simulink model "two_parallel_full_model_simscape"  (R2023b)
settings: Solver=ode1be  StartTime=0.0  StopTime=simlength  FixedStep=ts_sim  MaxStep=ts_sim
undefined symbols (not defined in the file): fclock, fPWM_INV, fPWM_ZVS, gate_nominal_voltage, I_FS, Iout_dc_nom, ki_i_inv, ki_i_zvs, ki_v_inv, ki_v_zvs, kp_i_inv, kp_i_zvs, kp_v_inv, kp_v_zvs, LFi_dc, LFu_ac, magnitude, n10, omega_grid, RCFu_dc, RLFi_dc, RLFu_ac, tc, Tc, tPWM_ZVS, ts_afe, ts_inv, ts_zvs, ugrid_factor, Ugrid_phase_normalization_factor, un_eta_pu, un_xi_pu, up_xi_pu, v1_trafo, v2_trafo, V_FS, Vout_dc_nom
libraries: fl_lib x142, nesl_utility x55, single_phase_transformer_lib x4
(part 1 of 4)
settings Model: SimulationMode=accelerator  Creator=LTNBDA  LastModifiedBy=dbagn
settings SolverCC: ZeroCrossControl=EnableAll  ZeroCrossAlgorithm=Adaptive  AlgebraicLoopSolver=TrustRegion  SolverResetMethod=Robust  AutoInsertRateTranBlk=on
settings DataIOCC: LimitDataPoints=on  MaxDataPoints=1  SaveFormat=Array  SignalLoggingSaveFormat=ModelDataLogs  SaveOutput=off  SignalLogging=off  DSMLogging=off  SaveTime=off  ReturnWorkspaceOutputs=off
settings OptimizationCC: ExpressionDepthLimit=2147483647  InitFltsAndDblsToZero=on  EfficientMapNaN2IntZero=off  LifeSpan=inf
settings DebuggingCC: SaveWithParameterizedLinksMsg=none  UnderspecifiedInitializationDetection=Classic  MergeDetectMultiDrivingBlocksExec=none  SignalResolutionControl=TryResolveAllWithWarning  SolverPrmCheckMsg=warning  MultiTaskDSMMsg=warning  MultiTaskCondExecSysMsg=none  MultiTaskRateTransMsg=warning  FcnCallInpInsideContextMsg=warning  StateNameClashWarn=warning  SFUnexpectedBacktrackingDiag=warning  SFNoUnconditionalDefaultTransitionDiag=warning  ArithmeticOperatorsInVariantConditions=warning
settings HardwareCC: ProdBitPerLong=64  ProdLargestAtomicFloat=None  ProdIntDivRoundTo=Undefined  ProdEndianess=Unspecified  ProdHWDeviceType=Generic->64-bit Embedded Processor (LP64)  TargetBitPerPointer=64  TargetBitPerSizeT=64  TargetBitPerPtrDiffT=64  TargetLongLongMode=on  TargetIntDivRoundTo=Zero  TargetEndianess=LittleEndian  TargetWordSize=64  TargetHWDeviceType=MATLAB Host  ProdEqTarget=off
settings ModelReferenceCC: EnableRefExpFcnMdlSchedulingChecks=on  PropagateSignalLabelsOutOfModel=off
settings SFSimCC: SimUseLocalCustomCode=off  CustomCodeUndefinedFunction=UseInterfaceOnly
settings RTWCC: RTWUseLocalCustomCode=off
settings CodeAppCC: MaxIdLength=128  StateflowObjectComments=on
settings GRTTargetCC: TargetLangStandard=C89/C90 (ANSI)  CombineOutputUpdateFcns=off  GRTInterface=on
settings ConfigComp: CovMetricSettings=dw  CovSaveCumulativeToWorkspaceVar=on  CovSaveSingleToWorkspaceVar=on  CovExternalEMLEnable=off
settings SimscapeCC: SimscapeNormalizeSystem=off

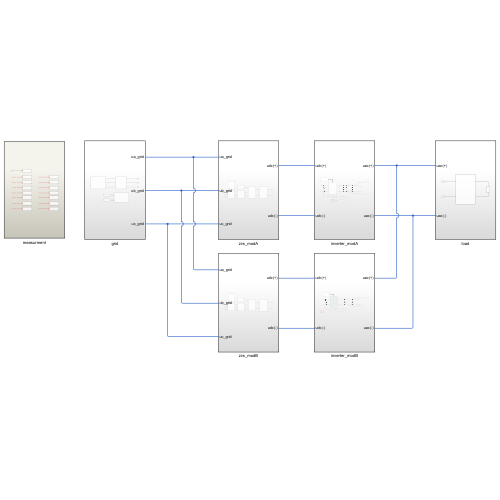
[thumbnail: Simulink's stored preview of the top-level diagram]
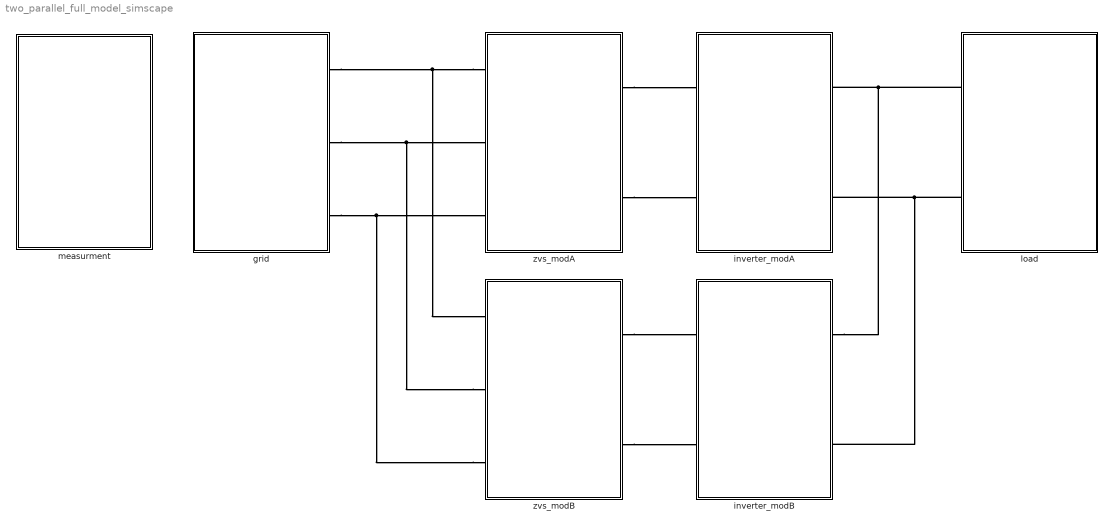
== system two_parallel_full_model_simscape ==
  grid : Subsystem
  inverter_modA : Subsystem
  inverter_modB : Subsystem
  load : Subsystem
  measurment : Subsystem
  zvs_modA : Subsystem
  zvs_modB : Subsystem
  connections:
  load/LConn1 -- inverter_modB/RConn1 -- inverter_modA/RConn1
  load/LConn2 -- inverter_modB/RConn2 -- inverter_modA/RConn2
  zvs_modA/LConn1 -- grid/RConn1 -- zvs_modB/LConn1
  zvs_modB/LConn2 -- grid/RConn2 -- zvs_modA/LConn2
  zvs_modB/LConn3 -- grid/RConn3 -- zvs_modA/LConn3
  zvs_modA/RConn2 -- inverter_modA/LConn2
  zvs_modA/RConn1 -- inverter_modA/LConn1
  zvs_modB/RConn1 -- inverter_modB/LConn1
  zvs_modB/RConn2 -- inverter_modB/LConn2

== system two_parallel_full_model_simscape/grid ==
  grid_emulator : Subsystem
  instantaneus_power : Subsystem
  threephase_vi_measures : Subsystem
  ua_grid : PMIOPort  Side=Right
  ub_grid : PMIOPort  Port=2  Side=Right
  uc_grid : PMIOPort  Port=3  Side=Right
  wires:
  [vg_abc] -> instantaneus_power/1(Vline)
  [ig_abc] -> instantaneus_power/2(Iline)
  connections:
  threephase_vi_measures/LConn3 -- grid_emulator/RConn3
  threephase_vi_measures/LConn2 -- grid_emulator/RConn2
  threephase_vi_measures/RConn1 -- ua_grid/RConn1
  threephase_vi_measures/LConn1 -- grid_emulator/RConn1
  threephase_vi_measures/RConn3 -- uc_grid/RConn1
  threephase_vi_measures/RConn2 -- ub_grid/RConn1

== system two_parallel_full_model_simscape/inverter_modA ==
  1/Ti3 : Gain  Gain=1/V_FS  SaturateOnIntegerOverflow=on  OutDataTypeStr=Inherit: Same as input  ParamDataTypeStr=Inherit: Same as input
  CFu_ac : fl_lib/Electrical/Electrical Elements/Capacitor  c=CFu_ac F  r=RCFu_ac Ohm  g=0 1/Ohm  i_specify=off  i_priority=None  i=0 A  i_nominal_specify=off  i_nominal_unit=A  i_nominal_value=1  v_specify=off  v_priority=None  v=0 V  v_nominal_specify=off  v_nominal_unit=V  v_nominal_value=1  vc_specify=off  vc_priority=High  vc=0 V  vc_nominal_specify=off  vc_nominal_unit=V  vc_nominal_value=1
  Current Sensor : fl_lib/Electrical/Electrical Sensors/Current Sensor
  Inductor1 : fl_lib/Electrical/Electrical Elements/Inductor  l=Lp H  r=0 Ohm  g=1e-9 1/Ohm  i_specify=off  i_priority=None  i=0 A  i_nominal_specify=off  i_nominal_unit=A  i_nominal_value=1  v_specify=off  v_priority=None  v=0 V  v_nominal_specify=off  v_nominal_unit=V  v_nominal_value=1  i_L_specify=off  i_L_priority=High  i_L=0 A  i_L_nominal_specify=off  i_L_nominal_unit=A  i_L_nominal_value=1
  Inductor2 : fl_lib/Electrical/Electrical Elements/Inductor  l=Lp H  r=0 Ohm  g=1e-9 1/Ohm  i_specify=off  i_priority=None  i=0 A  i_nominal_specify=off  i_nominal_unit=A  i_nominal_value=1  v_specify=off  v_priority=None  v=0 V  v_nominal_specify=off  v_nominal_unit=V  v_nominal_value=1  i_L_specify=off  i_L_priority=High  i_L=0 A  i_L_nominal_specify=off  i_L_nominal_unit=A  i_L_nominal_value=1
  LFu_ac_1 : fl_lib/Electrical/Electrical Elements/Inductor  l=LFu_ac/2 H  r=RLFu_ac/2 Ohm  g=0 1/Ohm  i_specify=off  i_priority=None  i=0 A  i_nominal_specify=off  i_nominal_unit=A  i_nominal_value=1  v_specify=off  v_priority=None  v=0 V  v_nominal_specify=off  v_nominal_unit=V  v_nominal_value=1  i_L_specify=off  i_L_priority=High  i_L=0 A  i_L_nominal_specify=off  i_L_nominal_unit=A  i_L_nominal_value=1
  LFu_ac_2 : fl_lib/Electrical/Electrical Elements/Inductor  l=LFu_ac/2 H  r=RLFu_ac/2 Ohm  g=0 1/Ohm  i_specify=off  i_priority=None  i=0 A  i_nominal_specify=off  i_nominal_unit=A  i_nominal_value=1  v_specify=off  v_priority=None  v=0 V  v_nominal_specify=off  v_nominal_unit=V  v_nominal_value=1  i_L_specify=off  i_L_priority=High  i_L=0 A  i_L_nominal_specify=off  i_L_nominal_unit=A  i_L_nominal_value=1
  Resistor : fl_lib/Electrical/Electrical Elements/Resistor  R=10e3 Ohm  i_specify=off  i_priority=None  i=0 A  i_nominal_specify=off  i_nominal_unit=A  i_nominal_value=1  v_specify=off  v_priority=None  v=0 V  v_nominal_specify=off  v_nominal_unit=V  v_nominal_value=1
  Voltage Sensor : fl_lib/Electrical/Electrical Sensors/Voltage Sensor
  Voltage Sensor1 : fl_lib/Electrical/Electrical Sensors/Voltage Sensor
  Zero-Order Hold2 : ZeroOrderHold  SampleTime=ts_zvs
  iph : nesl_utility/PS-Simulink Converter  PhysicalDomain=network_engine_domain  SubClassName=ps_output  LeftPortType=input  RightPortType=output  PseudoPeriodic=off  Frequencies=[]  VectorFormat=1-D array  Unit=A  AffineConversion=off
  phase_gen : Subsystem
  single phase inverter : Subsystem
      settings: PortSchema="{\"entries\":[{\"content\":{\"sides\":[{\"content\":{\"connectorIds\":[\"LConn1\",\"LConn2\"]},\"type\":\"ConnectorPlacement.EquallySpacedRectSide\",\"uuid\":\"4fcf4fea-d38f-431b-8a91-be3ce9782faf\"},{\"content\":{\"connectorIds\":[\"RConn1\",\"RConn2\"],\"side\":\"RIGHT\"},\"type\":\"ConnectorPlacement.EquallySpacedRectSide\",\"uuid\":\"0aa56277-92e9-4e3b-84c7-43398254a4d8\"},{\"content\":{\"connectorIds\":[\"In1\"],\"side\":\"TOP\"},\"type\":\"ConnectorPlacement.EquallySpacedRectSide\",\"uuid\":\"5cd150dc-bcaf-4cd7-b2a8-3db203726730\"}]},\"type\":\"ConnectorPlacement.EquallySpacedConnector\",\"uuid\":\"bf8194c4-c327-4d40-bea4-f1e7617f80b4\"}],\"packageUris\":[\"http://schema.mathworks.com/mf0/Connector/R2020b\"],\"version\":\"1.0\"}"
  single phase inverter control : Subsystem
  uph : nesl_utility/PS-Simulink Converter  PhysicalDomain=network_engine_domain  SubClassName=ps_output  LeftPortType=input  RightPortType=output  PseudoPeriodic=off  Frequencies=[]  VectorFormat=1-D array  Unit=V  AffineConversion=off
  uph1 : nesl_utility/PS-Simulink Converter  PhysicalDomain=network_engine_domain  SubClassName=ps_output  LeftPortType=input  RightPortType=output  PseudoPeriodic=off  Frequencies=[]  VectorFormat=1-D array  Unit=V  AffineConversion=off
  uac(+) : PMIOPort  Side=Right
  uac(-) : PMIOPort  Port=2  Side=Right
  udc(+) : PMIOPort  Port=3  Side=Left
  udc(-) : PMIOPort  Port=4  Side=Left
  tag scope: dclink_voltage_modA=global, inverter_current_output_modA=global, inverter_voltager_output_modA=global, phase_synch_modA=global
  wires:
  Zero-Order Hold2/1 -> 1/Ti3/1
  1/Ti3/1 -> [dclink_voltage_modA]
  single phase inverter control/1(gate_commands) -> single phase inverter/1(gate_commands)
  uph/1 -> Zero-Order Hold2/1  "uph"
  iph/1 -> [inverter_current_output_modA]  "iph"
  uph1/1 -> [inverter_voltager_output_modA]  "uph"
  phase_gen/1(emu_phase) -> [phase_synch_modA]
  connections:
  single phase inverter/RConn2 -- Voltage Sensor/RConn2 -- udc(-)/RConn1
  single phase inverter/RConn1 -- Voltage Sensor/LConn1 -- udc(+)/RConn1
  LFu_ac_1/LConn1 -- single phase inverter/LConn1
  Inductor1/RConn1 -- Voltage Sensor1/LConn1 -- Current Sensor/LConn1
  single phase inverter/LConn2 -- LFu_ac_2/RConn1
  LFu_ac_2/LConn1 -- Inductor2/LConn1 -- Resistor/RConn1 -- CFu_ac/RConn1
  Voltage Sensor/RConn1 -- uph/LConn1
  Voltage Sensor1/RConn1 -- uph1/LConn1
  Current Sensor/RConn1 -- iph/LConn1
  Voltage Sensor1/RConn2 -- Inductor2/RConn1 -- uac(-)/RConn1
  CFu_ac/LConn1 -- Inductor1/LConn1 -- Resistor/LConn1 -- LFu_ac_1/RConn1
  Current Sensor/RConn2 -- uac(+)/RConn1

== system two_parallel_full_model_simscape/inverter_modB ==
  1/Ti3 : Gain  Gain=1/V_FS  SaturateOnIntegerOverflow=on  OutDataTypeStr=Inherit: Same as input  ParamDataTypeStr=Inherit: Same as input
  CFu_ac : fl_lib/Electrical/Electrical Elements/Capacitor  c=CFu_ac F  r=RCFu_ac Ohm  g=0 1/Ohm  i_specify=off  i_priority=None  i=0 A  i_nominal_specify=off  i_nominal_unit=A  i_nominal_value=1  v_specify=off  v_priority=None  v=0 V  v_nominal_specify=off  v_nominal_unit=V  v_nominal_value=1  vc_specify=off  vc_priority=High  vc=0 V  vc_nominal_specify=off  vc_nominal_unit=V  vc_nominal_value=1
  Current Sensor : fl_lib/Electrical/Electrical Sensors/Current Sensor
  Inductor : fl_lib/Electrical/Electrical Elements/Inductor  l=Lp H  r=0 Ohm  g=1e-9 1/Ohm  i_specify=off  i_priority=None  i=0 A  i_nominal_specify=off  i_nominal_unit=A  i_nominal_value=1  v_specify=off  v_priority=None  v=0 V  v_nominal_specify=off  v_nominal_unit=V  v_nominal_value=1  i_L_specify=off  i_L_priority=High  i_L=0 A  i_L_nominal_specify=off  i_L_nominal_unit=A  i_L_nominal_value=1
  Inductor1 : fl_lib/Electrical/Electrical Elements/Inductor  l=Lp H  r=0 Ohm  g=1e-9 1/Ohm  i_specify=off  i_priority=None  i=0 A  i_nominal_specify=off  i_nominal_unit=A  i_nominal_value=1  v_specify=off  v_priority=None  v=0 V  v_nominal_specify=off  v_nominal_unit=V  v_nominal_value=1  i_L_specify=off  i_L_priority=High  i_L=0 A  i_L_nominal_specify=off  i_L_nominal_unit=A  i_L_nominal_value=1
  LFu_ac_1 : fl_lib/Electrical/Electrical Elements/Inductor  l=LFu_ac/2 H  r=RLFu_ac/2 Ohm  g=0 1/Ohm  i_specify=off  i_priority=None  i=0 A  i_nominal_specify=off  i_nominal_unit=A  i_nominal_value=1  v_specify=off  v_priority=None  v=0 V  v_nominal_specify=off  v_nominal_unit=V  v_nominal_value=1  i_L_specify=off  i_L_priority=High  i_L=0 A  i_L_nominal_specify=off  i_L_nominal_unit=A  i_L_nominal_value=1
  LFu_ac_2 : fl_lib/Electrical/Electrical Elements/Inductor  l=LFu_ac/2 H  r=RLFu_ac/2 Ohm  g=0 1/Ohm  i_specify=off  i_priority=None  i=0 A  i_nominal_specify=off  i_nominal_unit=A  i_nominal_value=1  v_specify=off  v_priority=None  v=0 V  v_nominal_specify=off  v_nominal_unit=V  v_nominal_value=1  i_L_specify=off  i_L_priority=High  i_L=0 A  i_L_nominal_specify=off  i_L_nominal_unit=A  i_L_nominal_value=1
  Resistor : fl_lib/Electrical/Electrical Elements/Resistor  R=10e3 Ohm  i_specify=off  i_priority=None  i=0 A  i_nominal_specify=off  i_nominal_unit=A  i_nominal_value=1  v_specify=off  v_priority=None  v=0 V  v_nominal_specify=off  v_nominal_unit=V  v_nominal_value=1
  Voltage Sensor : fl_lib/Electrical/Electrical Sensors/Voltage Sensor
  Voltage Sensor1 : fl_lib/Electrical/Electrical Sensors/Voltage Sensor
  Zero-Order Hold2 : ZeroOrderHold  SampleTime=ts_zvs
  iph : nesl_utility/PS-Simulink Converter  PhysicalDomain=network_engine_domain  SubClassName=ps_output  LeftPortType=input  RightPortType=output  PseudoPeriodic=off  Frequencies=[]  VectorFormat=1-D array  Unit=A  AffineConversion=off
  phase_gen : Subsystem
  single phase inverter : Subsystem
      settings: PortSchema="{\"entries\":[{\"content\":{\"sides\":[{\"content\":{\"connectorIds\":[\"LConn1\",\"LConn2\"]},\"type\":\"ConnectorPlacement.EquallySpacedRectSide\",\"uuid\":\"4fcf4fea-d38f-431b-8a91-be3ce9782faf\"},{\"content\":{\"connectorIds\":[\"RConn1\",\"RConn2\"],\"side\":\"RIGHT\"},\"type\":\"ConnectorPlacement.EquallySpacedRectSide\",\"uuid\":\"0aa56277-92e9-4e3b-84c7-43398254a4d8\"},{\"content\":{\"connectorIds\":[\"In1\"],\"side\":\"TOP\"},\"type\":\"ConnectorPlacement.EquallySpacedRectSide\",\"uuid\":\"5cd150dc-bcaf-4cd7-b2a8-3db203726730\"}]},\"type\":\"ConnectorPlacement.EquallySpacedConnector\",\"uuid\":\"bf8194c4-c327-4d40-bea4-f1e7617f80b4\"}],\"packageUris\":[\"http://schema.mathworks.com/mf0/Connector/R2020b\"],\"version\":\"1.0\"}"
  single phase inverter control : Subsystem
  uph : nesl_utility/PS-Simulink Converter  PhysicalDomain=network_engine_domain  SubClassName=ps_output  LeftPortType=input  RightPortType=output  PseudoPeriodic=off  Frequencies=[]  VectorFormat=1-D array  Unit=V  AffineConversion=off
  uph1 : nesl_utility/PS-Simulink Converter  PhysicalDomain=network_engine_domain  SubClassName=ps_output  LeftPortType=input  RightPortType=output  PseudoPeriodic=off  Frequencies=[]  VectorFormat=1-D array  Unit=V  AffineConversion=off
  uac(+) : PMIOPort  Side=Right
  uac(-) : PMIOPort  Port=2  Side=Right
  udc(+) : PMIOPort  Port=3  Side=Left
  udc(-) : PMIOPort  Port=4  Side=Left
  tag scope: dclink_voltage_modB=global, inverter_current_output_modB=global, inverter_voltager_output_modB=global, phase_synch_modB=global
  wires:
  uph1/1 -> [inverter_voltager_output_modB]  "uph"
  iph/1 -> [inverter_current_output_modB]  "iph"
  uph/1 -> Zero-Order Hold2/1  "uph"
  single phase inverter control/1(gate_commands) -> single phase inverter/1(gate_commands)
  1/Ti3/1 -> [dclink_voltage_modB]
  Zero-Order Hold2/1 -> 1/Ti3/1
  [gamma] -> [phase_synch_modB]
  connections:
  Current Sensor/RConn1 -- iph/LConn1
  Voltage Sensor1/RConn1 -- uph1/LConn1
  Voltage Sensor/RConn1 -- uph/LConn1
  Voltage Sensor1/RConn2 -- Inductor1/RConn1 -- uac(-)/RConn1
  single phase inverter/LConn2 -- LFu_ac_2/RConn1
  Inductor/RConn1 -- Voltage Sensor1/LConn1 -- Current Sensor/LConn1
  LFu_ac_1/LConn1 -- single phase inverter/LConn1
  Voltage Sensor/LConn1 -- single phase inverter/RConn1 -- udc(+)/RConn1
  Voltage Sensor/RConn2 -- udc(-)/RConn1 -- single phase inverter/RConn2
  Resistor/LConn1 -- CFu_ac/LConn1 -- LFu_ac_1/RConn1 -- Inductor/LConn1
  Resistor/RConn1 -- Inductor1/LConn1 -- LFu_ac_2/LConn1 -- CFu_ac/RConn1
  Current Sensor/RConn2 -- uac(+)/RConn1

== system two_parallel_full_model_simscape/load ==
  RL-load : fl_lib/Electrical/Electrical Elements/Inductor  l=Lload H  r=Rload Ohm  g=0 1/Ohm  i_specify=off  i_priority=None  i=0 A  i_nominal_specify=off  i_nominal_unit=A  i_nominal_value=1  v_specify=off  v_priority=None  v=0 V  v_nominal_specify=off  v_nominal_unit=V  v_nominal_value=1  i_L_specify=off  i_L_priority=High  i_L=0 A  i_L_nominal_specify=off  i_L_nominal_unit=A  i_L_nominal_value=1
  single_phase_ui_measure : Subsystem
  uac(+) : PMIOPort  Side=Left
  uac(-) : PMIOPort  Port=2  Side=Left
  connections:
  single_phase_ui_measure/LConn1 -- uac(+)/RConn1
  uac(-)/RConn1 -- single_phase_ui_measure/LConn2
  single_phase_ui_measure/RConn1 -- RL-load/LConn1
  RL-load/RConn1 -- single_phase_ui_measure/RConn2

== system two_parallel_full_model_simscape/measurment ==
  Clock : Clock
  To Workspace1 : ToWorkspace  VariableName=t  SampleTime=tc
      settings: MaxDataPoints=Nc
  To Workspace10 : ToWorkspace  Commented=on  VariableName=vi_CFu_ac  SampleTime=tc
      settings: MaxDataPoints=Nc
  To Workspace11 : ToWorkspace  Commented=on  VariableName=vi_LFu_ac  SampleTime=tc
      settings: MaxDataPoints=Nc
  To Workspace12 : ToWorkspace  Commented=on  VariableName=vi_LFi_dc  SampleTime=tc
      settings: MaxDataPoints=Nc
  To Workspace13 : ToWorkspace  Commented=on  VariableName=vi_Ls  SampleTime=tc
      settings: MaxDataPoints=Nc
  To Workspace14 : ToWorkspace  Commented=on  VariableName=vi_CFi_dc  SampleTime=tc
      settings: MaxDataPoints=Nc
  To Workspace15 : ToWorkspace  Commented=on  VariableName=i_d_rect  SampleTime=tc
      settings: MaxDataPoints=Nc
  To Workspace2 : ToWorkspace  Commented=on  VariableName=vi_RCFu_dc  SampleTime=tc
      settings: MaxDataPoints=Nc
  To Workspace3 : ToWorkspace  Commented=on  VariableName=vi_LFu_dc  SampleTime=tc
      settings: MaxDataPoints=Nc
  To Workspace4 : ToWorkspace  Commented=on  VariableName=vi_Cs  SampleTime=tc
      settings: MaxDataPoints=Nc
  To Workspace5 : ToWorkspace  Commented=on  VariableName=vi_load  SampleTime=tc
      settings: MaxDataPoints=Nc
  To Workspace6 : ToWorkspace  Commented=on  VariableName=vi_CFu_dc  SampleTime=tc
      settings: MaxDataPoints=Nc
  To Workspace7 : ToWorkspace  Commented=on  VariableName=vdc_in  SampleTime=tc
      settings: MaxDataPoints=Nc
  To Workspace8 : ToWorkspace  Commented=on  VariableName=Isnubber_H  SampleTime=tc
      settings: MaxDataPoints=Nc
  To Workspace9 : ToWorkspace  Commented=on  VariableName=Isnubber_Rect1  SampleTime=tc
      settings: MaxDataPoints=Nc
  wires:
  Clock/1 -> To Workspace1/1
  ? -> To Workspace3/1
  ? -> To Workspace6/1
  ? -> To Workspace2/1
  ? -> To Workspace4/1
  ? -> To Workspace5/1
  ? -> To Workspace7/1
  ? -> To Workspace8/1
  ? -> To Workspace9/1
  ? -> To Workspace11/1
  ? -> To Workspace10/1
  ? -> To Workspace12/1
  ? -> To Workspace13/1
  ? -> To Workspace14/1
  ? -> To Workspace15/1

== system two_parallel_full_model_simscape/zvs_modA ==
  dc/dc with galvanic isolation : Subsystem
  grid_rectifier : Subsystem
  measurment : Subsystem  Commented=on
  single_phase_ui_measure : Subsystem
  three_phase_vi_measures : Subsystem
  zvs_ctrl : Subsystem
  ua_grid : PMIOPort  Side=Left
  ub_grid : PMIOPort  Port=2  Side=Left
  uc_grid : PMIOPort  Port=3  Side=Left
  udc(+) : PMIOPort  Port=4  Side=Right
  udc(-) : PMIOPort  Port=5  Side=Right
  wires:
  zvs_ctrl/1(gate_commands) -> dc/dc with galvanic isolation/1(gate_commands)
  connections:
  grid_rectifier/LConn1 -- three_phase_vi_measures/RConn1
  grid_rectifier/LConn2 -- three_phase_vi_measures/RConn2
  grid_rectifier/LConn3 -- three_phase_vi_measures/RConn3
  ua_grid/RConn1 -- three_phase_vi_measures/LConn1
  ub_grid/RConn1 -- three_phase_vi_measures/LConn2
  uc_grid/RConn1 -- three_phase_vi_measures/LConn3
  dc/dc with galvanic isolation/LConn1 -- grid_rectifier/RConn1
  dc/dc with galvanic isolation/LConn2 -- grid_rectifier/RConn2
  dc/dc with galvanic isolation/RConn1 -- single_phase_ui_measure/LConn1
  dc/dc with galvanic isolation/RConn2 -- single_phase_ui_measure/LConn2
  udc(+)/RConn1 -- single_phase_ui_measure/RConn1
  udc(-)/RConn1 -- single_phase_ui_measure/RConn2

== system two_parallel_full_model_simscape/zvs_modB ==
  dc/dc with galvanic isolation : Subsystem
  grid_rectifier : Subsystem
  measurment : Subsystem  Commented=on
  single_phase_ui_measure : Subsystem
  three_phase_vi_measures : Subsystem
  zvs_ctrl : Subsystem
  ua_grid : PMIOPort  Side=Left
  ub_grid : PMIOPort  Port=2  Side=Left
  uc_grid : PMIOPort  Port=3  Side=Left
  udc(+) : PMIOPort  Port=4  Side=Right
  udc(-) : PMIOPort  Port=5  Side=Right
  wires:
  zvs_ctrl/1(gate_commands) -> dc/dc with galvanic isolation/1(gate_commands)
  connections:
  udc(-)/RConn1 -- single_phase_ui_measure/RConn2
  udc(+)/RConn1 -- single_phase_ui_measure/RConn1
  dc/dc with galvanic isolation/RConn2 -- single_phase_ui_measure/LConn2
  dc/dc with galvanic isolation/RConn1 -- single_phase_ui_measure/LConn1
  dc/dc with galvanic isolation/LConn2 -- grid_rectifier/RConn2
  dc/dc with galvanic isolation/LConn1 -- grid_rectifier/RConn1
  uc_grid/RConn1 -- three_phase_vi_measures/LConn3
  ub_grid/RConn1 -- three_phase_vi_measures/LConn2
  ua_grid/RConn1 -- three_phase_vi_measures/LConn1
  grid_rectifier/LConn3 -- three_phase_vi_measures/RConn3
  grid_rectifier/LConn2 -- three_phase_vi_measures/RConn2
  grid_rectifier/LConn1 -- three_phase_vi_measures/RConn1

== system two_parallel_full_model_simscape/grid/grid_emulator ==
  Controlled Voltage Source : fl_lib/Electrical/Electrical Sources/Controlled Voltage Source
  Controlled Voltage Source1 : fl_lib/Electrical/Electrical Sources/Controlled Voltage Source
  Controlled Voltage Source2 : fl_lib/Electrical/Electrical Sources/Controlled Voltage Source
  Electrical Reference : fl_lib/Electrical/Electrical Elements/Electrical Reference
  Ld2_grid_1 : fl_lib/Electrical/Electrical Elements/Inductor  l=60e-6 H  r=5e-3 Ohm  g=1e-9 1/Ohm  i_specify=on  i_priority=High  i=0 A  i_nominal_specify=off  i_nominal_unit=A  i_nominal_value=1  v_specify=off  v_priority=None  v=0 V  v_nominal_specify=off  v_nominal_unit=V  v_nominal_value=1  i_L_specify=off  i_L_priority=High  i_L=0 A  i_L_nominal_specify=off  i_L_nominal_unit=A  i_L_nominal_value=1
  Ld2_grid_2 : fl_lib/Electrical/Electrical Elements/Inductor  l=60e-6 H  r=5e-3 Ohm  g=1e-9 1/Ohm  i_specify=on  i_priority=High  i=0 A  i_nominal_specify=off  i_nominal_unit=A  i_nominal_value=1  v_specify=off  v_priority=None  v=0 V  v_nominal_specify=off  v_nominal_unit=V  v_nominal_value=1  i_L_specify=off  i_L_priority=High  i_L=0 A  i_L_nominal_specify=off  i_L_nominal_unit=A  i_L_nominal_value=1
  Ld2_grid_3 : fl_lib/Electrical/Electrical Elements/Inductor  l=60e-6 H  r=5e-3 Ohm  g=1e-9 1/Ohm  i_specify=on  i_priority=High  i=0 A  i_nominal_specify=off  i_nominal_unit=A  i_nominal_value=1  v_specify=off  v_priority=None  v=0 V  v_nominal_specify=off  v_nominal_unit=V  v_nominal_value=1  i_L_specify=off  i_L_priority=High  i_L=0 A  i_L_nominal_specify=off  i_L_nominal_unit=A  i_L_nominal_value=1
  Simulink-PS Converter : nesl_utility/Simulink-PS Converter  PhysicalDomain=network_engine_domain  SubClassName=ps_input  LeftPortType=input  RightPortType=output  PseudoPeriodic=off  Frequencies=[]  NoiseDistribution=none  NoiseParameters=[]  Unit=V  AffineConversion=on  FilteringAndDerivatives=provide  SimscapeFilterOrder=1  InputFilterTimeConstant=0.001  UdotUserProvided=0
  Simulink-PS Converter1 : nesl_utility/Simulink-PS Converter  PhysicalDomain=network_engine_domain  SubClassName=ps_input  LeftPortType=input  RightPortType=output  PseudoPeriodic=off  Frequencies=[]  NoiseDistribution=none  NoiseParameters=[]  Unit=V  AffineConversion=on  FilteringAndDerivatives=provide  SimscapeFilterOrder=1  InputFilterTimeConstant=0.001  UdotUserProvided=0
  Simulink-PS Converter2 : nesl_utility/Simulink-PS Converter  PhysicalDomain=network_engine_domain  SubClassName=ps_input  LeftPortType=input  RightPortType=output  PseudoPeriodic=off  Frequencies=[]  NoiseDistribution=none  NoiseParameters=[]  Unit=V  AffineConversion=on  FilteringAndDerivatives=provide  SimscapeFilterOrder=1  InputFilterTimeConstant=0.001  UdotUserProvided=0
  Solver Configuration : nesl_utility/Solver Configuration  PhysicalDomain=network_engine_domain  SubClassName=solver  LeftPortType=input  RightPortType=generic  Tones=[]  Harmonics=[]  SimulateNoise=off  Profile=off  UseLocalSampling=off  EnableSwitchedLinearOptims=on  FrequencyDomain=off  UseCCode=off  RelTol=0.001  AbsTol=0.001  MinStep=1e-09  ToWorkspace=off  RevertToSquareIcSolve=off  NumHomotopyIterations=100  PhasorMode=off  PhasorModeNumHarmonics=1  ConsistencySolver=NEWTON_FTOL  IndexReductionMethod=DerivativeReplacement  DoDC=on  ResidualTolerance=1e-09  ConsistencyTolSource=GLOBAL  ConsistencyAbsTol=0.001  ConsistencyRelTol=0.001  ConsistencyTolFactor=0.001  UseLocalSolver=on  LocalSolverChoice=NE_BACKWARD_EULER_ADVANCER  ResolveIndetEquations=on  FunctionEvalNumThread=1  LocalSolverSampleTime=ts_sim  DoFixedCost=on  MaxNonlinIter=3  MaxModeIter=2  ComputeImpulses=off  ImpulseIterations=2  LinearAlgebra=auto  LinearAlgebraNumThread=0  EquationFormulation=NE_TIME_EF  DelaysMemoryBudget=1024  AutomaticFiltering=on  FilteringTimeConstant=0.001  PartitionStorageMethod=AS_NEEDED  PartitionMemoryBudget=1024  PartitionMethod=ROBUST  MultibodyUseLocalSolver=off  MultibodyLocalSolverChoice=ODE1  MultibodyLocalSolverSampleTime=0.001
  grid_source : Subsystem
  ua_grid : PMIOPort  Side=Right
  ub_grid : PMIOPort  Port=2  Side=Right
  uc_grid : PMIOPort  Port=3  Side=Right
  wires:
  grid_source/2(us_grid) -> Simulink-PS Converter1/1
  grid_source/3(ut_grid) -> Simulink-PS Converter2/1
  grid_source/1(ur_grid) -> Simulink-PS Converter/1
  connections:
  Simulink-PS Converter/RConn1 -- Controlled Voltage Source/RConn1
  Simulink-PS Converter1/RConn1 -- Controlled Voltage Source1/RConn1
  Simulink-PS Converter2/RConn1 -- Controlled Voltage Source2/RConn1
  Electrical Reference/LConn1 -- Solver Configuration/RConn1 -- Controlled Voltage Source/RConn2 -- Controlled Voltage Source1/RConn2 -- Controlled Voltage Source2/RConn2
  Ld2_grid_1/LConn1 -- Controlled Voltage Source/LConn1
  ub_grid/RConn1 -- Ld2_grid_2/RConn1
  Ld2_grid_3/LConn1 -- Controlled Voltage Source2/LConn1
  ua_grid/RConn1 -- Ld2_grid_1/RConn1
  Ld2_grid_2/LConn1 -- Controlled Voltage Source1/LConn1
  uc_grid/RConn1 -- Ld2_grid_3/RConn1

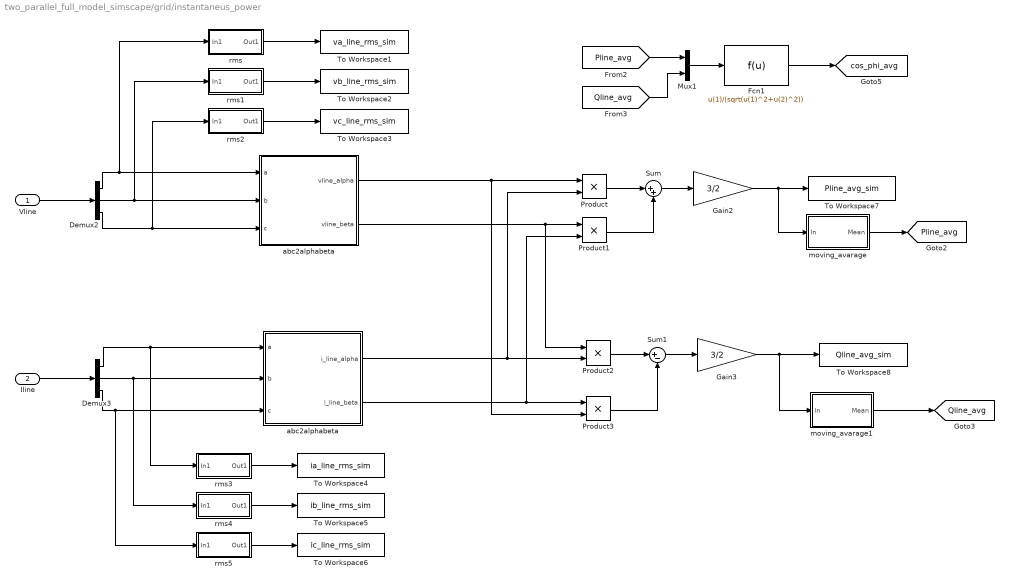
== system two_parallel_full_model_simscape/grid/instantaneus_power ==
  Vline : Inport
  Iline : Inport  Port=2
  Demux2 : Demux  Outputs=3
  Demux3 : Demux  Outputs=3
  Fcn1 : Fcn  Expr=u(1)/(sqrt(u(1)^2+u(2)^2))
  Gain2 : Gain  Gain=3/2
  Gain3 : Gain  Gain=3/2
  Mux1 : Mux  Inputs=2
  Product{,1..3} (4 alike) : Product  RndMeth=Zero
  Sum : Sum  Inputs=|++
  Sum1 : Sum  Inputs=|+-
  To Workspace1 : ToWorkspace  VariableName=va_line_rms_sim  SampleTime=ts_afe
      settings: MaxDataPoints=Ns_afe
  To Workspace2 : ToWorkspace  VariableName=vb_line_rms_sim  SampleTime=ts_afe
      settings: MaxDataPoints=Ns_afe
  To Workspace3 : ToWorkspace  VariableName=vc_line_rms_sim  SampleTime=ts_afe
      settings: MaxDataPoints=Ns_afe
  To Workspace4 : ToWorkspace  VariableName=ia_line_rms_sim  SampleTime=ts_afe
      settings: MaxDataPoints=Ns_afe
  To Workspace5 : ToWorkspace  VariableName=ib_line_rms_sim  SampleTime=ts_afe
      settings: MaxDataPoints=Ns_afe
  To Workspace6 : ToWorkspace  VariableName=ic_line_rms_sim  SampleTime=ts_afe
      settings: MaxDataPoints=Ns_afe
  To Workspace7 : ToWorkspace  VariableName=Pline_avg_sim  SampleTime=ts_afe
      settings: MaxDataPoints=Ns_afe
  To Workspace8 : ToWorkspace  VariableName=Qline_avg_sim  SampleTime=ts_afe
      settings: MaxDataPoints=Ns_afe
  abc2alphabeta : Subsystem
  "abc2alphabeta " : Subsystem
  moving_avarage : Subsystem
  moving_avarage1 : Subsystem
  rms : Subsystem
  rms1 : Subsystem
  rms2 : Subsystem
  rms3 : Subsystem
  rms4 : Subsystem
  rms5 : Subsystem
  tag scope: Pline_avg=global, Qline_avg=global, cos_phi_avg=global
  wires:
  Gain3/1 -> moving_avarage1/1(In), To Workspace8/1
  Gain2/1 -> moving_avarage/1(In), To Workspace7/1
  Demux2/1 -> abc2alphabeta/1(a), rms/1(In1)
  Vline/1 -> Demux2/1
  Iline/1 -> Demux3/1
  abc2alphabeta/2(vline_beta) -> Product1/1, Product2/1
  "abc2alphabeta "/2(i_line_beta) -> Product3/1, Product1/2
  abc2alphabeta/1(vline_alpha) -> Product/1, Product3/2
  "abc2alphabeta "/1(i_line_alpha) -> Product2/2, Product/2
  Product/1 -> Sum/1
  Product1/1 -> Sum/2
  Product2/1 -> Sum1/1
  Product3/1 -> Sum1/2
  Sum1/1 -> Gain3/1
  Sum/1 -> Gain2/1
  Demux2/2 -> abc2alphabeta/2(b), rms1/1(In1)
  Demux2/3 -> abc2alphabeta/3(c), rms2/1(In1)
  Demux3/1 -> "abc2alphabeta "/1(a), rms3/1(In1)
  Demux3/2 -> "abc2alphabeta "/2(b), rms4/1(In1)
  Demux3/3 -> rms5/1(In1), "abc2alphabeta "/3(c)
  moving_avarage/1(Mean) -> [Pline_avg]
  moving_avarage1/1(Mean) -> [Qline_avg]
  [Qline_avg] -> Mux1/2
  Mux1/1 -> Fcn1/1
  Fcn1/1 -> [cos_phi_avg]
  [Pline_avg] -> Mux1/1
  rms/1(Out1) -> To Workspace1/1
  rms2/1(Out1) -> To Workspace3/1
  rms1/1(Out1) -> To Workspace2/1
  rms5/1(Out1) -> To Workspace6/1
  rms4/1(Out1) -> To Workspace5/1
  rms3/1(Out1) -> To Workspace4/1

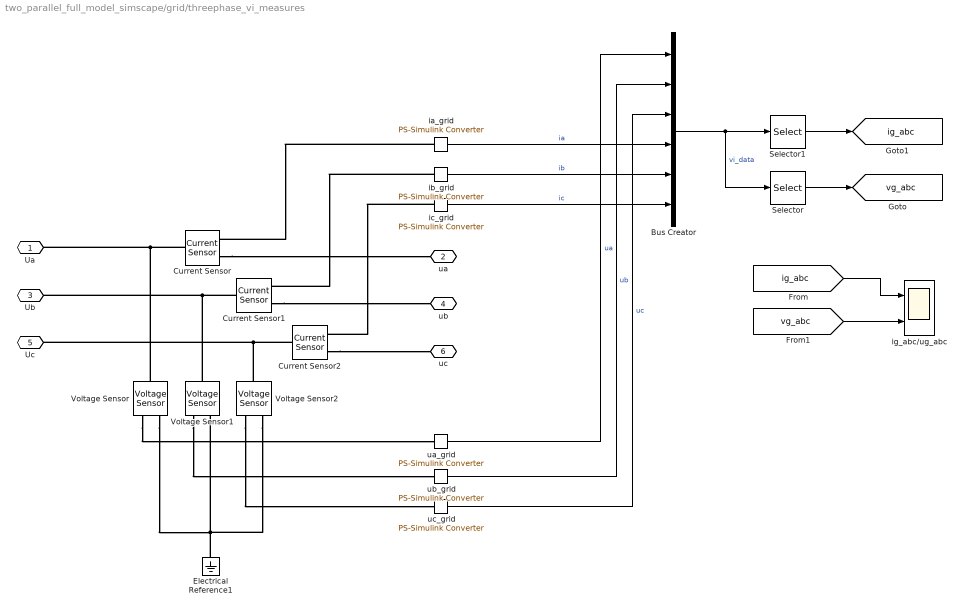
== system two_parallel_full_model_simscape/grid/threephase_vi_measures ==
  Bus Creator : BusCreator  Inputs=6
  Current Sensor : fl_lib/Electrical/Electrical Sensors/Current Sensor
  Current Sensor1 : fl_lib/Electrical/Electrical Sensors/Current Sensor
  Current Sensor2 : fl_lib/Electrical/Electrical Sensors/Current Sensor
  Electrical Reference1 : fl_lib/Electrical/Electrical Elements/Electrical Reference
  Selector : Selector  InputPortWidth=6  IndexOptions=Index vector (dialog)  Indices=[1 2 3]  OutputSizes=1
  Selector1 : Selector  InputPortWidth=6  IndexOptions=Index vector (dialog)  Indices=[4 5 6]  OutputSizes=1
  Voltage Sensor : fl_lib/Electrical/Electrical Sensors/Voltage Sensor
  Voltage Sensor1 : fl_lib/Electrical/Electrical Sensors/Voltage Sensor
  Voltage Sensor2 : fl_lib/Electrical/Electrical Sensors/Voltage Sensor
  ia_grid : nesl_utility/PS-Simulink Converter  PhysicalDomain=network_engine_domain  SubClassName=ps_output  LeftPortType=input  RightPortType=output  PseudoPeriodic=off  Frequencies=[]  VectorFormat=1-D array  Unit=A  AffineConversion=off
  ib_grid : nesl_utility/PS-Simulink Converter  PhysicalDomain=network_engine_domain  SubClassName=ps_output  LeftPortType=input  RightPortType=output  PseudoPeriodic=off  Frequencies=[]  VectorFormat=1-D array  Unit=A  AffineConversion=off
  ic_grid : nesl_utility/PS-Simulink Converter  PhysicalDomain=network_engine_domain  SubClassName=ps_output  LeftPortType=input  RightPortType=output  PseudoPeriodic=off  Frequencies=[]  VectorFormat=1-D array  Unit=A  AffineConversion=off
  ig_abc/ug_abc : Scope  NumInputPorts=2
  ua_grid : nesl_utility/PS-Simulink Converter  PhysicalDomain=network_engine_domain  SubClassName=ps_output  LeftPortType=input  RightPortType=output  PseudoPeriodic=off  Frequencies=[]  VectorFormat=1-D array  Unit=V  AffineConversion=off
  ub_grid : nesl_utility/PS-Simulink Converter  PhysicalDomain=network_engine_domain  SubClassName=ps_output  LeftPortType=input  RightPortType=output  PseudoPeriodic=off  Frequencies=[]  VectorFormat=1-D array  Unit=V  AffineConversion=off
  uc_grid : nesl_utility/PS-Simulink Converter  PhysicalDomain=network_engine_domain  SubClassName=ps_output  LeftPortType=input  RightPortType=output  PseudoPeriodic=off  Frequencies=[]  VectorFormat=1-D array  Unit=V  AffineConversion=off
  Ua : PMIOPort  Side=Left
  ua : PMIOPort  Port=2  Side=Right
  Ub : PMIOPort  Port=3  Side=Left
  ub : PMIOPort  Port=4  Side=Right
  Uc : PMIOPort  Port=5  Side=Left
  uc : PMIOPort  Port=6  Side=Right
  tag scope: ig_abc=global, vg_abc=global
  wires:
  Bus Creator/1 -> Selector1/1, Selector/1  "vi_data"
  Selector/1 -> [vg_abc]
  ib_grid/1 -> Bus Creator/5  "ib"
  ia_grid/1 -> Bus Creator/4  "ia"
  ic_grid/1 -> Bus Creator/6  "ic"
  ua_grid/1 -> Bus Creator/1  "ua"
  ub_grid/1 -> Bus Creator/2  "ub"
  uc_grid/1 -> Bus Creator/3  "uc"
  Selector1/1 -> [ig_abc]
  [vg_abc] -> ig_abc/ug_abc/2
  [ig_abc] -> ig_abc/ug_abc/1
  connections:
  Current Sensor1/LConn1 -- Ub/RConn1 -- Voltage Sensor1/LConn1
  Electrical Reference1/LConn1 -- Voltage Sensor/RConn2 -- Voltage Sensor2/RConn2 -- Voltage Sensor1/RConn2
  Voltage Sensor/RConn1 -- ua_grid/LConn1
  Current Sensor/RConn2 -- ua/RConn1
  Voltage Sensor1/RConn1 -- ub_grid/LConn1
  Voltage Sensor2/LConn1 -- Current Sensor2/LConn1 -- Uc/RConn1
  Current Sensor/LConn1 -- Ua/RConn1 -- Voltage Sensor/LConn1
  Current Sensor1/RConn2 -- ub/RConn1
  Voltage Sensor2/RConn1 -- uc_grid/LConn1
  ib_grid/LConn1 -- Current Sensor1/RConn1
  ia_grid/LConn1 -- Current Sensor/RConn1
  ic_grid/LConn1 -- Current Sensor2/RConn1
  Current Sensor2/RConn2 -- uc/RConn1

== system two_parallel_full_model_simscape/inverter_modA/phase_gen ==
  Constant4 : Constant  Value=omega_grid
  Integrator : Integrator
  bounder1 : MATLAB Function  TreatAsAtomicUnit=on  SystemSampleTime=ts_afe
  emu_phase : Outport  VectorParamsAs1DForOutWhenUnconnected=off
  tag scope: gamma=global
  wires:
  bounder1/1(y) -> [gamma], emu_phase/1  "emu_phase"
  Constant4/1 -> Integrator/1
  Integrator/1 -> bounder1/1(u)

== system two_parallel_full_model_simscape/inverter_modA/single phase inverter ==
  gate_commands : Inport
  Bus Selector : BusSelector  OutputSignals=gate_cmd_Q1 (signal 1),gate_cmd_Q2 (signal 2),gate_cmd_Q1 (signal 3),gate_cmd_Q2 (signal 4)
  Simulink-PS Converter{,1..3} (4 alike) : nesl_utility/Simulink-PS Converter  PhysicalDomain=network_engine_domain  SubClassName=ps_input  LeftPortType=input  RightPortType=output  PseudoPeriodic=off  Frequencies=[]  NoiseDistribution=none  NoiseParameters=[]  Unit=1  AffineConversion=on  FilteringAndDerivatives=provide  SimscapeFilterOrder=1  InputFilterTimeConstant=0.001  UdotUserProvided=0
  switch_1 : Subsystem
      settings: PortSchema="{\"entries\":[{\"content\":{\"sides\":[{\"content\":{\"connectorIds\":[\"LConn1\"]},\"type\":\"ConnectorPlacement.EquallySpacedRectSide\",\"uuid\":\"9277da8d-d460-43e6-8478-dd662f15d226\"},{\"content\":{\"connectorIds\":[],\"side\":\"RIGHT\"},\"type\":\"ConnectorPlacement.EquallySpacedRectSide\",\"uuid\":\"a7ece396-f1d9-4f4f-a05b-db1fc65d6e1d\"},{\"content\":{\"connectorIds\":[\"LConn2\"],\"side\":\"TOP\"},\"type\":\"ConnectorPlacement.EquallySpacedRectSide\",\"uuid\":\"fdd70777-e9cf-4317-afb6-cae87f75d5b0\"},{\"content\":{\"connectorIds\":[\"RConn1\"],\"side\":\"BOTTOM\"},\"type\":\"ConnectorPlacement.EquallySpacedRectSide\",\"uuid\":\"2353ed68-b1a1-4775-9ca9-31e268d5443b\"}]},\"type\":\"ConnectorPlacement.EquallySpacedConnector\",\"uuid\":\"d5479f4c-4e65-4791-adcb-73df11f88590\"}],\"packageUris\":[\"http://schema.mathworks.com/mf0/Connector/R2020b\"],\"version\":\"1.0\"}"
  switch_2 : Subsystem
      settings: PortSchema="{\"entries\":[{\"content\":{\"sides\":[{\"content\":{\"connectorIds\":[\"LConn1\"]},\"type\":\"ConnectorPlacement.EquallySpacedRectSide\",\"uuid\":\"9277da8d-d460-43e6-8478-dd662f15d226\"},{\"content\":{\"connectorIds\":[],\"side\":\"RIGHT\"},\"type\":\"ConnectorPlacement.EquallySpacedRectSide\",\"uuid\":\"a7ece396-f1d9-4f4f-a05b-db1fc65d6e1d\"},{\"content\":{\"connectorIds\":[\"LConn2\"],\"side\":\"TOP\"},\"type\":\"ConnectorPlacement.EquallySpacedRectSide\",\"uuid\":\"fdd70777-e9cf-4317-afb6-cae87f75d5b0\"},{\"content\":{\"connectorIds\":[\"RConn1\"],\"side\":\"BOTTOM\"},\"type\":\"ConnectorPlacement.EquallySpacedRectSide\",\"uuid\":\"2353ed68-b1a1-4775-9ca9-31e268d5443b\"}]},\"type\":\"ConnectorPlacement.EquallySpacedConnector\",\"uuid\":\"d5479f4c-4e65-4791-adcb-73df11f88590\"}],\"packageUris\":[\"http://schema.mathworks.com/mf0/Connector/R2020b\"],\"version\":\"1.0\"}"
  switch_3 : Subsystem
      settings: PortSchema="{\"entries\":[{\"content\":{\"sides\":[{\"content\":{\"connectorIds\":[\"LConn1\"]},\"type\":\"ConnectorPlacement.EquallySpacedRectSide\",\"uuid\":\"9277da8d-d460-43e6-8478-dd662f15d226\"},{\"content\":{\"connectorIds\":[],\"side\":\"RIGHT\"},\"type\":\"ConnectorPlacement.EquallySpacedRectSide\",\"uuid\":\"a7ece396-f1d9-4f4f-a05b-db1fc65d6e1d\"},{\"content\":{\"connectorIds\":[\"LConn2\"],\"side\":\"TOP\"},\"type\":\"ConnectorPlacement.EquallySpacedRectSide\",\"uuid\":\"fdd70777-e9cf-4317-afb6-cae87f75d5b0\"},{\"content\":{\"connectorIds\":[\"RConn1\"],\"side\":\"BOTTOM\"},\"type\":\"ConnectorPlacement.EquallySpacedRectSide\",\"uuid\":\"2353ed68-b1a1-4775-9ca9-31e268d5443b\"}]},\"type\":\"ConnectorPlacement.EquallySpacedConnector\",\"uuid\":\"d5479f4c-4e65-4791-adcb-73df11f88590\"}],\"packageUris\":[\"http://schema.mathworks.com/mf0/Connector/R2020b\"],\"version\":\"1.0\"}"
  switch_4 : Subsystem
      settings: PortSchema="{\"entries\":[{\"content\":{\"sides\":[{\"content\":{\"connectorIds\":[\"LConn1\"]},\"type\":\"ConnectorPlacement.EquallySpacedRectSide\",\"uuid\":\"9277da8d-d460-43e6-8478-dd662f15d226\"},{\"content\":{\"connectorIds\":[],\"side\":\"RIGHT\"},\"type\":\"ConnectorPlacement.EquallySpacedRectSide\",\"uuid\":\"a7ece396-f1d9-4f4f-a05b-db1fc65d6e1d\"},{\"content\":{\"connectorIds\":[\"LConn2\"],\"side\":\"TOP\"},\"type\":\"ConnectorPlacement.EquallySpacedRectSide\",\"uuid\":\"fdd70777-e9cf-4317-afb6-cae87f75d5b0\"},{\"content\":{\"connectorIds\":[\"RConn1\"],\"side\":\"BOTTOM\"},\"type\":\"ConnectorPlacement.EquallySpacedRectSide\",\"uuid\":\"2353ed68-b1a1-4775-9ca9-31e268d5443b\"}]},\"type\":\"ConnectorPlacement.EquallySpacedConnector\",\"uuid\":\"d5479f4c-4e65-4791-adcb-73df11f88590\"}],\"packageUris\":[\"http://schema.mathworks.com/mf0/Connector/R2020b\"],\"version\":\"1.0\"}"
  uac_out(+) : PMIOPort  Side=Left
  uac_out(-) : PMIOPort  Port=2  Side=Left
  udc(+) : PMIOPort  Port=3  Side=Right
  udc(-) : PMIOPort  Port=4  Side=Right
  wires:
  [gate_Q1] -> Simulink-PS Converter/1
  [gate_Q2] -> Simulink-PS Converter1/1
  [gate_Q3] -> Simulink-PS Converter2/1
  [gate_Q4] -> Simulink-PS Converter3/1
  gate_commands/1 -> Bus Selector/1
  Bus Selector/1 -> [gate_Q1]  "<gate_cmd_Q1 (signal 1)>"
  Bus Selector/2 -> [gate_Q2]  "<gate_cmd_Q2 (signal 2)>"
  Bus Selector/3 -> [gate_Q3]  "<gate_cmd_Q1 (signal 3)>"
  Bus Selector/4 -> [gate_Q4]  "<gate_cmd_Q2 (signal 4)>"
  connections:
  switch_3/LConn2 -- switch_1/LConn2 -- udc(+)/RConn1
  udc(-)/RConn1 -- switch_4/RConn1 -- switch_2/RConn1
  Simulink-PS Converter/RConn1 -- switch_1/LConn1
  switch_2/LConn1 -- Simulink-PS Converter1/RConn1
  switch_3/LConn1 -- Simulink-PS Converter2/RConn1
  switch_4/LConn1 -- Simulink-PS Converter3/RConn1
  uac_out(+)/RConn1 -- switch_2/LConn2 -- switch_1/RConn1
  uac_out(-)/RConn1 -- switch_4/LConn2 -- switch_3/RConn1

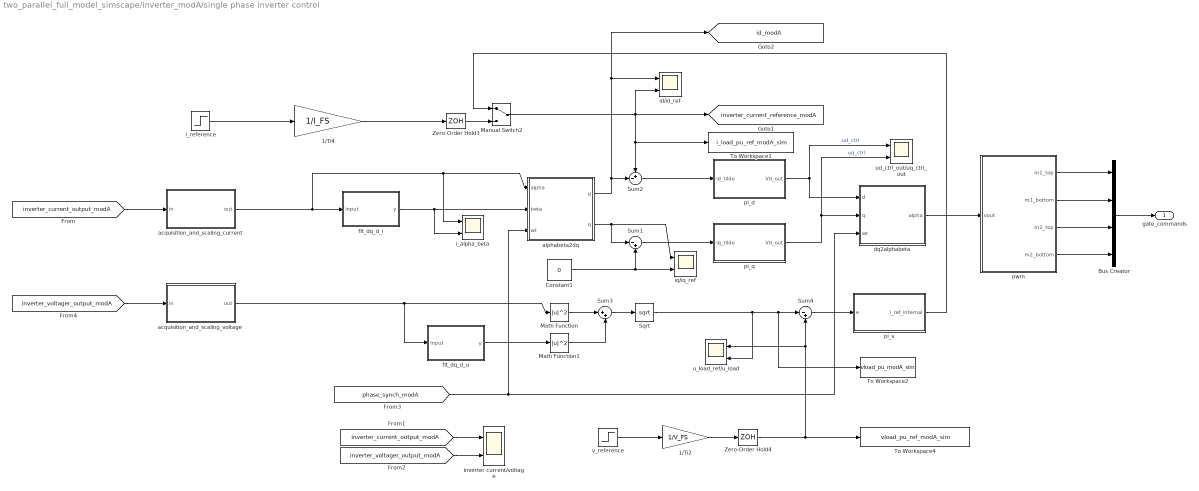
== system two_parallel_full_model_simscape/inverter_modA/single phase inverter control ==
  1/Ti2 : Gain  Gain=1/V_FS  SaturateOnIntegerOverflow=on  OutDataTypeStr=Inherit: Same as input  ParamDataTypeStr=Inherit: Same as input
  1/Ti4 : Gain  Gain=1/I_FS  SaturateOnIntegerOverflow=on  OutDataTypeStr=Inherit: Same as input  ParamDataTypeStr=Inherit: Same as input
  Bus Creator : BusCreator  Inputs=4
  Constant1 : Constant  Value=0
  Manual Switch2 : ManualSwitch
  Math Function : Math  Operator=magnitude^2
  Math Function1 : Math  Operator=magnitude^2
  Sqrt : Sqrt
  Sum1 : Sum  Inputs=|-+
  Sum2 : Sum  Inputs=+-|
  Sum3 : Sum  Inputs=|++
  Sum4 : Sum  Inputs=|-+
  To Workspace1 : ToWorkspace  VariableName=i_load_pu_ref_modA_sim  SampleTime=ts_inv
      settings: MaxDataPoints=Ns_inv
  To Workspace2 : ToWorkspace  VariableName=vload_pu_modA_sim  SampleTime=ts_inv
      settings: MaxDataPoints=Ns_inv
  To Workspace4 : ToWorkspace  VariableName=vload_pu_ref_modA_sim  SampleTime=ts_inv
      settings: MaxDataPoints=Ns_inv
  Zero-Order Hold3 : ZeroOrderHold  SampleTime=ts_inv
  Zero-Order Hold4 : ZeroOrderHold  SampleTime=ts_inv
  acquisition_and_scaling_current : Subsystem
  acquisition_and_scaling_voltage : Subsystem
  alphabeta2dq : Subsystem
  dq2alphabeta : Subsystem
  flt_dq_d_i : MATLAB Function  TreatAsAtomicUnit=on  SystemSampleTime=ts_inv
  flt_dq_d_u : MATLAB Function  TreatAsAtomicUnit=on  SystemSampleTime=ts_inv
  i_alpha_beta : Scope  NumInputPorts=2
  i_reference : Step  Time=0.1  After=55*sqrt(2)  SampleTime=0
  id/id_ref : Scope  NumInputPorts=2
  inverter current/voltage : Scope  NumInputPorts=2
  iq/iq_ref : Scope  NumInputPorts=2
  pi_d : Subsystem
  pi_q : Subsystem
  pi_v : Subsystem
  pwm : Subsystem
  u_load_ref/u_load : Scope  NumInputPorts=2
  ud_ctrl_out/uq_ctrl_out : Scope  NumInputPorts=2
  v_reference : Step  After=500*sqrt(2)  SampleTime=0
  gate_commands : Outport
  tag scope: id_modA=global, inverter_current_reference_modA=global
  wires:
  dq2alphabeta/1(alpha) -> pwm/1(vout)
  i_reference/1 -> 1/Ti4/1
  1/Ti4/1 -> Zero-Order Hold3/1
  flt_dq_d_i/1(y) -> i_alpha_beta/2, alphabeta2dq/2(beta)
  [phase_synch_modA] -> alphabeta2dq/3(wt), dq2alphabeta/3(wt)
  alphabeta2dq/2("q ") -> Sum1/1, iq/iq_ref/1
  alphabeta2dq/1("d ") -> [id_modA], id/id_ref/1, Sum2/2
  Zero-Order Hold3/1 -> Manual Switch2/2
  Manual Switch2/1 -> id/id_ref/2, [inverter_current_reference_modA], Sum2/1, To Workspace1/1
  Constant1/1 -> iq/iq_ref/2, Sum1/2
  Sum2/1 -> pi_d/1(id_tilde)
  Sum1/1 -> pi_q/1(iq_tilde)
  pi_d/1(Vd_out) -> ud_ctrl_out/uq_ctrl_out/1, dq2alphabeta/1(d)  "ud_ctrl"
  pi_q/1(Vd_out) -> dq2alphabeta/2(q), ud_ctrl_out/uq_ctrl_out/2  "uq_ctrl"
  flt_dq_d_u/1(y) -> Math Function1/1
  Math Function/1 -> Sum3/1
  Math Function1/1 -> Sum3/2
  Sum3/1 -> Sqrt/1
  1/Ti2/1 -> Zero-Order Hold4/1
  v_reference/1 -> 1/Ti2/1
  Sqrt/1 -> u_load_ref/u_load/2, To Workspace2/1, Sum4/1
  Zero-Order Hold4/1 -> Sum4/2, u_load_ref/u_load/1, To Workspace4/1
  Sum4/1 -> pi_v/1(e)
  pi_v/1(i_ref_internal) -> Manual Switch2/1
  pwm/3(m2_top) -> Bus Creator/3
  Bus Creator/1 -> gate_commands/1
  pwm/1(m1_top) -> Bus Creator/1
  pwm/2(m1_bottom) -> Bus Creator/2
  pwm/4(m2_bottom) -> Bus Creator/4
  acquisition_and_scaling_current/1(out) -> flt_dq_d_i/1(input), i_alpha_beta/1, alphabeta2dq/1(alpha)
  [inverter_current_output_modA] -> acquisition_and_scaling_current/1(in)
  acquisition_and_scaling_voltage/1(out) -> flt_dq_d_u/1(input), Math Function/1
  [inverter_voltager_output_modA] -> acquisition_and_scaling_voltage/1(in)
  [inverter_current_output_modA] -> inverter current/voltage/1
  [inverter_voltager_output_modA] -> inverter current/voltage/2

== system two_parallel_full_model_simscape/inverter_modB/phase_gen ==
  Constant4 : Constant  Value=omega_grid
  Integrator : Integrator
  bounder1 : MATLAB Function  TreatAsAtomicUnit=on  SystemSampleTime=ts_afe
  emu_phase : Outport  VectorParamsAs1DForOutWhenUnconnected=off
  wires:
  bounder1/1(y) -> emu_phase/1  "emu_phase"
  Constant4/1 -> Integrator/1
  Integrator/1 -> bounder1/1(u)

== system two_parallel_full_model_simscape/inverter_modB/single phase inverter ==
  gate_commands : Inport
  Bus Selector : BusSelector  OutputSignals=gate_cmd_Q1 (signal 1),gate_cmd_Q2 (signal 2),gate_cmd_Q1 (signal 3),gate_cmd_Q2 (signal 4)
  Simulink-PS Converter{,1..3} (4 alike) : nesl_utility/Simulink-PS Converter  PhysicalDomain=network_engine_domain  SubClassName=ps_input  LeftPortType=input  RightPortType=output  PseudoPeriodic=off  Frequencies=[]  NoiseDistribution=none  NoiseParameters=[]  Unit=1  AffineConversion=on  FilteringAndDerivatives=provide  SimscapeFilterOrder=1  InputFilterTimeConstant=0.001  UdotUserProvided=0
  switch_1 : Subsystem
      settings: PortSchema="{\"entries\":[{\"content\":{\"sides\":[{\"content\":{\"connectorIds\":[\"LConn1\"]},\"type\":\"ConnectorPlacement.EquallySpacedRectSide\",\"uuid\":\"9277da8d-d460-43e6-8478-dd662f15d226\"},{\"content\":{\"connectorIds\":[],\"side\":\"RIGHT\"},\"type\":\"ConnectorPlacement.EquallySpacedRectSide\",\"uuid\":\"a7ece396-f1d9-4f4f-a05b-db1fc65d6e1d\"},{\"content\":{\"connectorIds\":[\"LConn2\"],\"side\":\"TOP\"},\"type\":\"ConnectorPlacement.EquallySpacedRectSide\",\"uuid\":\"fdd70777-e9cf-4317-afb6-cae87f75d5b0\"},{\"content\":{\"connectorIds\":[\"RConn1\"],\"side\":\"BOTTOM\"},\"type\":\"ConnectorPlacement.EquallySpacedRectSide\",\"uuid\":\"2353ed68-b1a1-4775-9ca9-31e268d5443b\"}]},\"type\":\"ConnectorPlacement.EquallySpacedConnector\",\"uuid\":\"d5479f4c-4e65-4791-adcb-73df11f88590\"}],\"packageUris\":[\"http://schema.mathworks.com/mf0/Connector/R2020b\"],\"version\":\"1.0\"}"
  switch_2 : Subsystem
      settings: PortSchema="{\"entries\":[{\"content\":{\"sides\":[{\"content\":{\"connectorIds\":[\"LConn1\"]},\"type\":\"ConnectorPlacement.EquallySpacedRectSide\",\"uuid\":\"9277da8d-d460-43e6-8478-dd662f15d226\"},{\"content\":{\"connectorIds\":[],\"side\":\"RIGHT\"},\"type\":\"ConnectorPlacement.EquallySpacedRectSide\",\"uuid\":\"a7ece396-f1d9-4f4f-a05b-db1fc65d6e1d\"},{\"content\":{\"connectorIds\":[\"LConn2\"],\"side\":\"TOP\"},\"type\":\"ConnectorPlacement.EquallySpacedRectSide\",\"uuid\":\"fdd70777-e9cf-4317-afb6-cae87f75d5b0\"},{\"content\":{\"connectorIds\":[\"RConn1\"],\"side\":\"BOTTOM\"},\"type\":\"ConnectorPlacement.EquallySpacedRectSide\",\"uuid\":\"2353ed68-b1a1-4775-9ca9-31e268d5443b\"}]},\"type\":\"ConnectorPlacement.EquallySpacedConnector\",\"uuid\":\"d5479f4c-4e65-4791-adcb-73df11f88590\"}],\"packageUris\":[\"http://schema.mathworks.com/mf0/Connector/R2020b\"],\"version\":\"1.0\"}"
  switch_3 : Subsystem
      settings: PortSchema="{\"entries\":[{\"content\":{\"sides\":[{\"content\":{\"connectorIds\":[\"LConn1\"]},\"type\":\"ConnectorPlacement.EquallySpacedRectSide\",\"uuid\":\"9277da8d-d460-43e6-8478-dd662f15d226\"},{\"content\":{\"connectorIds\":[],\"side\":\"RIGHT\"},\"type\":\"ConnectorPlacement.EquallySpacedRectSide\",\"uuid\":\"a7ece396-f1d9-4f4f-a05b-db1fc65d6e1d\"},{\"content\":{\"connectorIds\":[\"LConn2\"],\"side\":\"TOP\"},\"type\":\"ConnectorPlacement.EquallySpacedRectSide\",\"uuid\":\"fdd70777-e9cf-4317-afb6-cae87f75d5b0\"},{\"content\":{\"connectorIds\":[\"RConn1\"],\"side\":\"BOTTOM\"},\"type\":\"ConnectorPlacement.EquallySpacedRectSide\",\"uuid\":\"2353ed68-b1a1-4775-9ca9-31e268d5443b\"}]},\"type\":\"ConnectorPlacement.EquallySpacedConnector\",\"uuid\":\"d5479f4c-4e65-4791-adcb-73df11f88590\"}],\"packageUris\":[\"http://schema.mathworks.com/mf0/Connector/R2020b\"],\"version\":\"1.0\"}"
  switch_4 : Subsystem
      settings: PortSchema="{\"entries\":[{\"content\":{\"sides\":[{\"content\":{\"connectorIds\":[\"LConn1\"]},\"type\":\"ConnectorPlacement.EquallySpacedRectSide\",\"uuid\":\"9277da8d-d460-43e6-8478-dd662f15d226\"},{\"content\":{\"connectorIds\":[],\"side\":\"RIGHT\"},\"type\":\"ConnectorPlacement.EquallySpacedRectSide\",\"uuid\":\"a7ece396-f1d9-4f4f-a05b-db1fc65d6e1d\"},{\"content\":{\"connectorIds\":[\"LConn2\"],\"side\":\"TOP\"},\"type\":\"ConnectorPlacement.EquallySpacedRectSide\",\"uuid\":\"fdd70777-e9cf-4317-afb6-cae87f75d5b0\"},{\"content\":{\"connectorIds\":[\"RConn1\"],\"side\":\"BOTTOM\"},\"type\":\"ConnectorPlacement.EquallySpacedRectSide\",\"uuid\":\"2353ed68-b1a1-4775-9ca9-31e268d5443b\"}]},\"type\":\"ConnectorPlacement.EquallySpacedConnector\",\"uuid\":\"d5479f4c-4e65-4791-adcb-73df11f88590\"}],\"packageUris\":[\"http://schema.mathworks.com/mf0/Connector/R2020b\"],\"version\":\"1.0\"}"
  uac_out(+) : PMIOPort  Side=Left
  uac_out(-) : PMIOPort  Port=2  Side=Left
  udc(+) : PMIOPort  Port=3  Side=Right
  udc(-) : PMIOPort  Port=4  Side=Right
  wires:
  Bus Selector/4 -> [gate_Q4]  "<gate_cmd_Q2 (signal 4)>"
  Bus Selector/3 -> [gate_Q3]  "<gate_cmd_Q1 (signal 3)>"
  Bus Selector/2 -> [gate_Q2]  "<gate_cmd_Q2 (signal 2)>"
  Bus Selector/1 -> [gate_Q1]  "<gate_cmd_Q1 (signal 1)>"
  gate_commands/1 -> Bus Selector/1
  [gate_Q4] -> Simulink-PS Converter3/1
  [gate_Q3] -> Simulink-PS Converter2/1
  [gate_Q2] -> Simulink-PS Converter1/1
  [gate_Q1] -> Simulink-PS Converter/1
  connections:
  switch_3/RConn1 -- switch_4/LConn2 -- uac_out(-)/RConn1
  switch_1/RConn1 -- switch_2/LConn2 -- uac_out(+)/RConn1
  switch_4/LConn1 -- Simulink-PS Converter3/RConn1
  switch_3/LConn1 -- Simulink-PS Converter2/RConn1
  switch_2/LConn1 -- Simulink-PS Converter1/RConn1
  Simulink-PS Converter/RConn1 -- switch_1/LConn1
  switch_2/RConn1 -- switch_4/RConn1 -- udc(-)/RConn1
  udc(+)/RConn1 -- switch_1/LConn2 -- switch_3/LConn2

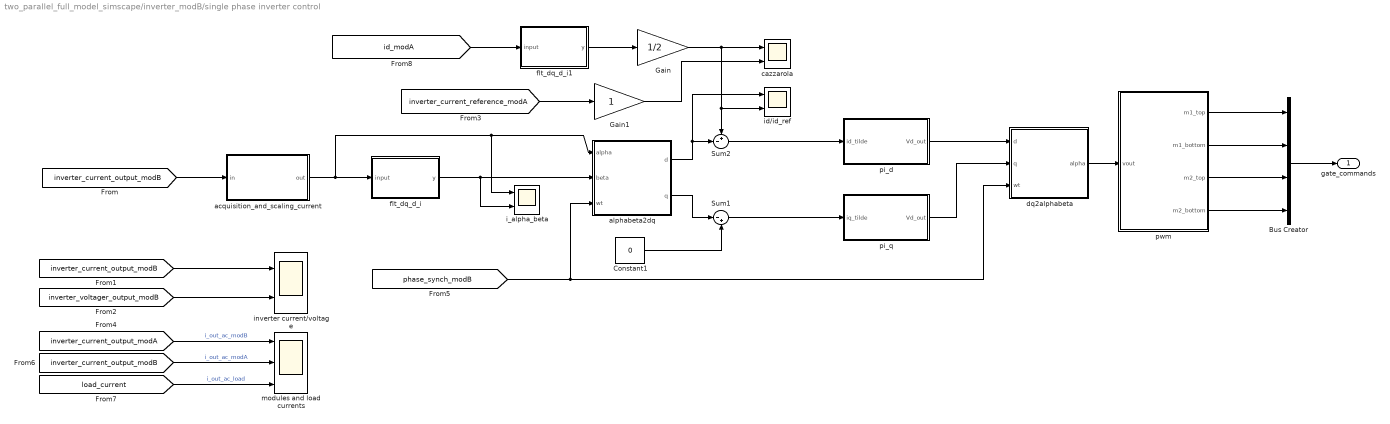
== system two_parallel_full_model_simscape/inverter_modB/single phase inverter control ==
  Bus Creator : BusCreator  Inputs=4
  Constant1 : Constant  Value=0
  Gain : Gain  Gain=1/2
  Gain1 : Gain
  Sum1 : Sum  Inputs=|-+
  Sum2 : Sum  Inputs=+-|
  acquisition_and_scaling_current : Subsystem
  alphabeta2dq : Subsystem
  cazzarola : Scope  NumInputPorts=2
  dq2alphabeta : Subsystem
  flt_dq_d_i : MATLAB Function  TreatAsAtomicUnit=on  SystemSampleTime=ts_inv
  flt_dq_d_i1 : MATLAB Function  TreatAsAtomicUnit=on  SystemSampleTime=ts_inv
  i_alpha_beta : Scope  NumInputPorts=2
  id/id_ref : Scope  NumInputPorts=2
  inverter current/voltage : Scope  NumInputPorts=2
  modules and load currents : Scope  NumInputPorts=3
  pi_d : Subsystem
  pi_q : Subsystem
  pwm : Subsystem
  gate_commands : Outport
  wires:
  [inverter_voltager_output_modB] -> inverter current/voltage/2
  [inverter_current_output_modB] -> inverter current/voltage/1
  [inverter_current_output_modB] -> acquisition_and_scaling_current/1(in)
  acquisition_and_scaling_current/1(out) -> alphabeta2dq/1(alpha), i_alpha_beta/1, flt_dq_d_i/1(input)
  [inverter_current_output_modB] -> modules and load currents/2  "i_out_ac_modA"
  [load_current] -> modules and load currents/3  "i_out_ac_load"
  [inverter_current_output_modA] -> modules and load currents/1  "i_out_ac_modB"
  pwm/4(m2_bottom) -> Bus Creator/4
  pwm/2(m1_bottom) -> Bus Creator/2
  pwm/1(m1_top) -> Bus Creator/1
  Bus Creator/1 -> gate_commands/1
  pwm/3(m2_top) -> Bus Creator/3
  pi_q/1(Vd_out) -> dq2alphabeta/2(q)
  pi_d/1(Vd_out) -> dq2alphabeta/1(d)
  Sum1/1 -> pi_q/1(iq_tilde)
  Sum2/1 -> pi_d/1(id_tilde)
  Constant1/1 -> Sum1/2
  alphabeta2dq/1("d ") -> id/id_ref/1, Sum2/2
  alphabeta2dq/2("q ") -> Sum1/1
  flt_dq_d_i/1(y) -> alphabeta2dq/2(beta), i_alpha_beta/2
  dq2alphabeta/1(alpha) -> pwm/1(vout)
  [phase_synch_modB] -> dq2alphabeta/3(wt), alphabeta2dq/3(wt)
  [id_modA] -> flt_dq_d_i1/1(input)
  flt_dq_d_i1/1(y) -> Gain/1
  Gain/1 -> Sum2/1, id/id_ref/2, cazzarola/1
  [inverter_current_reference_modA] -> Gain1/1
  Gain1/1 -> cazzarola/2
